simulink model "Collision_two_cars_cs"  (Simulink 8.7)
settings: Solver=ode5  SolverMode=SingleTasking  StartTime=0.0  StopTime=inf  FixedStep=1/20  RelTol=1e-3
model workspace (MAT data in the model file):
  mbox_table.block_array(1).src = 'built-in/Subsystem'
  mbox_table.block_array(1).dest = 'Collision_two_cars_cs/Audi_A8_1'
  mbox_table.block_array(1).mode = 0
  mbox_table.block_array(2).src = 'simulink/Sinks/Out1'
  mbox_table.block_array(2).dest = 'Collision_two_cars_cs/Audi_A8_1/STATE_Audi_A8_1'
  mbox_table.block_array(2).mode = 0
  mbox_table.block_array(3).src = 'PreScanSimulinkLibrary/State'
  mbox_table.block_array(3).dest = 'Collision_two_cars_cs/STATE_Audi_A8_1'
  mbox_table.block_array(3).mode = 0
  mbox_table.block_array(4).src = 'PreScanSimulinkLibrary/Trajectories'
  mbox_table.block_array(4).dest = 'Collision_two_cars_cs/Audi_A8_1/Trajectories'
  mbox_table.block_array(4).mode = 0
  mbox_table.block_array(5).src = 'simulink/Sources/Constant'
  mbox_table.block_array(5).dest = 'Collision_two_cars_cs/Audi_A8_1/Trajectories/Trajectory_1_Offset'
  mbox_table.block_array(5).mode = 0
  mbox_table.block_array(6).src = 'PreScanSimulinkLibrary/Trajectory'
  mbox_table.block_array(6).dest = 'Collision_two_cars_cs/Audi_A8_1/Trajectories/Trajectory_1'
  mbox_table.block_array(6).mode = 0
  mbox_table.block_array(7).src = 'PreScanSimulinkLibrary/Traj2State'
  mbox_table.block_array(7).dest = 'Collision_two_cars_cs/Audi_A8_1/Trajectories/Traj2State1'
  mbox_table.block_array(7).mode = 0
  mbox_table.block_array(8).src = 'simulink/Sinks/Out1'
  mbox_table.block_array(8).dest = 'Collision_two_cars_cs/Audi_A8_1/Trajectories/State'
  mbox_table.block_array(8).mode = 0
  mbox_table.block_array(9).src = 'PreScanSimulinkLibrary/SELF'
  mbox_table.block_array(9).dest = 'Collision_two_cars_cs/SELF_Audi_A8_1'
  mbox_table.block_array(9).mode = 0
  mbox_table.block_array(10).src = 'simulink/Sources/In1'
  mbox_table.block_array(10).dest = 'Collision_two_cars_cs/Audi_A8_1/SELF_Audi_A8_1'
  mbox_table.block_array(10).mode = 0
  mbox_table.block_array(11).src = 'PreScanSimulinkLibrary/DemuxSELF'
  mbox_table.block_array(11).dest = 'Collision_two_cars_cs/Audi_A8_1/SELF_Demux'
  mbox_table.block_array(11).mode = 0
  mbox_table.block_array(12).src = 'built-in/S-Function'
  mbox_table.block_array(12).dest = 'Collision_two_cars_cs/AIR_1'
  mbox_table.block_array(12).mode = 0
  mbox_table.block_array(13).src = 'simulink/Sources/In1'
  mbox_table.block_array(13).dest = 'Collision_two_cars_cs/Audi_A8_1/AIR_1'
  mbox_table.block_array(13).mode = 0
  mbox_table.block_array(14).src = 'PreScanSimulinkLibrary/DemuxAIR'
  mbox_table.block_array(14).dest = 'Collision_two_cars_cs/Audi_A8_1/AIR_1_Demux'
  mbox_table.block_array(14).mode = 0
  mbox_table.block_array(15).src = 'built-in/Subsystem'
  mbox_table.block_array(15).dest = 'Collision_two_cars_cs/BMW_X5_1'
  mbox_table.block_array(15).mode = 0
  mbox_table.block_array(16).src = 'simulink/Sinks/Out1'
  mbox_table.block_array(16).dest = 'Collision_two_cars_cs/BMW_X5_1/STATE_BMW_X5_1'
  mbox_table.block_array(16).mode = 0
  mbox_table.block_array(17).src = 'PreScanSimulinkLibrary/State'
  mbox_table.block_array(17).dest = 'Collision_two_cars_cs/STATE_BMW_X5_1'
  mbox_table.block_array(17).mode = 0
  mbox_table.block_array(18).src = 'PreScanSimulinkLibrary/Trajectories'
  mbox_table.block_array(18).dest = 'Collision_two_cars_cs/BMW_X5_1/Trajectories'
  mbox_table.block_array(18).mode = 0
  mbox_table.block_array(19).src = 'simulink/Sources/Constant'
  mbox_table.block_array(19).dest = 'Collision_two_cars_cs/BMW_X5_1/Trajectories/Trajectory_2_Offset'
  mbox_table.block_array(19).mode = 0
  mbox_table.block_array(20).src = 'PreScanSimulinkLibrary/Trajectory'
  mbox_table.block_array(20).dest = 'Collision_two_cars_cs/BMW_X5_1/Trajectories/Trajectory_2'
  mbox_table.block_array(20).mode = 0
  mbox_table.block_array(21).src = 'PreScanSimulinkLibrary/Traj2State'
  mbox_table.block_array(21).dest = 'Collision_two_cars_cs/BMW_X5_1/Trajectories/Traj2State1'
  mbox_table.block_array(21).mode = 0
  mbox_table.block_array(22).src = 'simulink/Sinks/Out1'
  mbox_table.block_array(22).dest = 'Collision_two_cars_cs/BMW_X5_1/Trajectories/State'
  mbox_table.block_array(22).mode = 0
  mbox_table.block_array(23).src = 'PreScanSimulinkLibrary/SELF'
  mbox_table.block_array(23).dest = 'Collision_two_cars_cs/SELF_BMW_X5_1'
  mbox_table.block_array(23).mode = 0
  mbox_table.block_array(24).src = 'simulink/Sources/In1'
  mbox_table.block_array(24).dest = 'Collision_two_cars_cs/BMW_X5_1/SELF_BMW_X5_1'
  mbox_table.block_array(24).mode = 0
  mbox_table.block_array(25).src = 'PreScanSimulinkLibrary/DemuxSELF'
  mbox_table.block_array(25).dest = 'Collision_two_cars_cs/BMW_X5_1/SELF_Demux'
  mbox_table.block_array(25).mode = 0
  mbox_table.block_array(26).src = 'SimCoreLibrary/SimCoreConfiguration'
  mbox_table.block_array(26).dest = 'Collision_two_cars_cs/SimCoreConfiguration'
  mbox_table.block_array(26).mode = 0
  mbox_table.block_array(27).src = 'SimCoreLibrary/Actuators'
  mbox_table.block_array(27).dest = 'Collision_two_cars_cs/Actuators'
  mbox_table.block_array(27).mode = 0
  mbox_table.block_array(28).src = 'SimCoreLibrary/SetActuators'
  mbox_table.block_array(28).dest = 'Collision_two_cars_cs/SetActuators'
  mbox_table.block_array(28).mode = 0
  mbox_table.block_array(29).src = 'SimCoreLibrary/GetSensors'
  mbox_table.block_array(29).dest = 'Collision_two_cars_cs/GetSensors'
  mbox_table.block_array(29).mode = 0
  mbox_table.block_array(30).src = 'SimCoreLibrary/SimCoreInfo'
  mbox_table.block_array(30).dest = 'Collision_two_cars_cs/SimCoreInfo'
  mbox_table.block_array(30).mode = 0
  mbox_table.block_array(31).src = 'PreScanSimulinkLibrary/Regenerate'
  mbox_table.block_array(31).dest = 'Collision_two_cars_cs/Regenerate'
  mbox_table.block_array(31).mode = 0
  mbox_table.block_array(32).src = 'PreScanSimulinkLibrary/Record for Replay  '
  mbox_table.block_array(32).dest = 'Collision_two_cars_cs/Record for Replay  '
  mbox_table.block_array(32).mode = 0
  mbox_table.block_array(33).src = 'PreScanSimulinkLibrary/Open Useful Blocks'
  mbox_table.block_array(33).dest = 'Collision_two_cars_cs/Open Useful Blocks'
  mbox_table.block_array(33).mode = 0
  mbox_table.block_array(34).src = 'PreScanSimulinkLibrary/PreScan Options   '
  mbox_table.block_array(34).dest = 'Collision_two_cars_cs/PreScan Options   '
  mbox_table.block_array(34).mode = 0
  mbox_table.block_array(35).src = 'built-in/Note'
  mbox_table.block_array(35).dest = 'Collision_two_cars_cs/Version:                  '
  mbox_table.block_array(35).mode = 0
  mbox_table.block_array(36).src = 'built-in/Note'
  mbox_table.block_array(36).dest = 'Collision_two_cars_cs/7.4.0'
  mbox_table.block_array(36).mode = 0
  mbox_table.block_array(37).src = 'built-in/Note'
  mbox_table.block_array(37).dest = 'Collision_two_cars_cs/Author(s):                '
  mbox_table.block_array(37).mode = 0
  mbox_table.block_array(38).src = 'built-in/Note'
  mbox_table.block_array(38).dest = 'Collision_two_cars_cs/Weikas'
  mbox_table.block_array(38).mode = 0
  mbox_table.block_array(39).src = 'built-in/Note'
  mbox_table.block_array(39).dest = 'Collision_two_cars_cs/Descriptive text:      '
  mbox_table.block_array(39).mode = 0
  mbox_table.block_array(40).src = 'built-in/Note'
  mbox_table.block_array(40).dest = 'Collision_two_cars_cs/Collision between two cars'
  mbox_table.block_array(40).mode = 0
  mbox_table.block_array(41).src = 'built-in/Note'
  mbox_table.block_array(41).dest = 'Collision_two_cars_cs/ID
    | 
    | 1
    | 2'
  mbox_table.block_array(41).mode = 0
  mbox_table.block_array(42).src = 'built-in/Note'
  mbox_table.block_array(42).dest = 'Collision_two_cars_cs/OBU-Beacon ID
    | 
    | 
    | '
  mbox_table.block_array(42).mode = 0
  mbox_table.block_array(43).src = 'built-in/Note'
  mbox_table.block_array(43).dest = 'Collision_two_cars_cs/TypeID
    | 
    | 1
    | 1'
  mbox_table.block_array(43).mode = 0
  mbox_table.block_array(44).src = 'built-in/Note'
  mbox_table.block_array(44).dest = 'Collision_two_cars_cs/TypeTag
    | 
    | Car
    | Car'
  mbox_table.block_array(44).mode = 0
  mbox_table.block_array(45).src = 'built-in/Note'
  mbox_table.block_array(45).dest = 'Collision_two_cars_cs/SD
    | 
    | Y
    | Y'
  mbox_table.block_array(45).mode = 0
  mbox_table.block_array(46).src = 'built-in/Note'
  mbox_table.block_array(46).dest = 'Collision_two_cars_cs/CD
    | 
    | N
    | N'
  mbox_table.block_array(46).mode = 0
  mbox_table.block_array(47).src = 'built-in/Note'
  mbox_table.block_array(47).dest = 'Collision_two_cars_cs/Name
    | 
    | Audi_A8_1
    | BMW_X5_1'
  mbox_table.block_array(47).mode = 0
  mbox_table.block_array(48).src = 'built-in/Note'
  mbox_table.block_array(48).dest = 'Collision_two_cars_cs/Num ID       OBU-Beacon ID     Type ID      Type Tag             SD        CD             Name                          '
  mbox_table.block_array(48).mode = 0
  mbox_table.block_array(49).src = 'built-in/Terminator'
  mbox_table.block_array(49).dest = 'Collision_two_cars_cs/BMW_X5_1/Terminator_1'
  mbox_table.block_array(49).mode = 1
  mbox_table.block_array(50).src = 'built-in/Terminator'
  mbox_table.block_array(50).dest = 'Collision_two_cars_cs/BMW_X5_1/Terminator_2'
  mbox_table.block_array(50).mode = 1
  mbox_table.block_array(51).src = 'built-in/Terminator'
  mbox_table.block_array(51).dest = 'Collision_two_cars_cs/BMW_X5_1/Terminator_3'
  mbox_table.block_array(51).mode = 1
  mbox_table.block_array(52).src = 'built-in/Terminator'
  mbox_table.block_array(52).dest = 'Collision_two_cars_cs/BMW_X5_1/Terminator_4'
  mbox_table.block_array(52).mode = 1
  mbox_table.block_array(53).src = 'built-in/Terminator'
  mbox_table.block_array(53).dest = 'Collision_two_cars_cs/BMW_X5_1/Terminator_5'
  mbox_table.block_array(53).mode = 1
  mbox_table.block_array(54).src = 'built-in/Terminator'
  mbox_table.block_array(54).dest = 'Collision_two_cars_cs/BMW_X5_1/Terminator_6'
  mbox_table.block_array(54).mode = 1
  mbox_table.block_array(55).src = 'built-in/Terminator'
  mbox_table.block_array(55).dest = 'Collision_two_cars_cs/BMW_X5_1/Terminator_7'
  mbox_table.block_array(55).mode = 1
  mbox_table.block_array(56).src = 'built-in/Terminator'
  mbox_table.block_array(56).dest = 'Collision_two_cars_cs/BMW_X5_1/Terminator_8'
  mbox_table.block_array(56).mode = 1
  mbox_table.block_array(57).src = 'built-in/Terminator'
  mbox_table.block_array(57).dest = 'Collision_two_cars_cs/BMW_X5_1/Terminator_9'
  mbox_table.block_array(57).mode = 1
  mbox_table.block_array(58).src = 'built-in/Terminator'
  mbox_table.block_array(58).dest = 'Collision_two_cars_cs/BMW_X5_1/Terminator_10'
  mbox_table.block_array(58).mode = 1
  mbox_table.block_array(59).src = 'built-in/Terminator'
  mbox_table.block_array(59).dest = 'Collision_two_cars_cs/BMW_X5_1/Terminator_11'
  mbox_table.block_array(59).mode = 1
  mbox_table.block_array(60).src = 'built-in/Terminator'
  mbox_table.block_array(60).dest = 'Collision_two_cars_cs/BMW_X5_1/Terminator_12'
  mbox_table.block_array(60).mode = 1
  mbox_table.block_index : java.util.Hashtable (value not decoded)
  mbox_table.line_array(1).sys = 'Collision_two_cars_cs'
  mbox_table.line_array(1).line_id = 'L1'
  mbox_table.line_array(1).iport = 'STATE_Audi_A8_1/1'
  mbox_table.line_array(1).oport = 'Audi_A8_1/1'
  mbox_table.line_array(1).mode = 0
  mbox_table.line_array(2).sys = 'Collision_two_cars_cs/Audi_A8_1/Trajectories'
  mbox_table.line_array(2).line_id = 'L2'
  mbox_table.line_array(2).iport = 'Traj2State1/1'
  mbox_table.line_array(2).oport = 'Trajectory_1/1'
  mbox_table.line_array(2).mode = 0
  mbox_table.line_array(3).sys = 'Collision_two_cars_cs/Audi_A8_1/Trajectories'
  mbox_table.line_array(3).line_id = 'L3'
  mbox_table.line_array(3).iport = 'Traj2State1/2'
  mbox_table.line_array(3).oport = 'Trajectory_1_Offset/1'
  mbox_table.line_array(3).mode = 0
  mbox_table.line_array(4).sys = 'Collision_two_cars_cs/Audi_A8_1/Trajectories'
  mbox_table.line_array(4).line_id = 'L4'
  mbox_table.line_array(4).iport = 'State/1'
  mbox_table.line_array(4).oport = 'Traj2State1/1'
  mbox_table.line_array(4).mode = 0
  mbox_table.line_array(5).sys = 'Collision_two_cars_cs'
  mbox_table.line_array(5).line_id = 'L5'
  mbox_table.line_array(5).iport = 'Audi_A8_1/1'
  mbox_table.line_array(5).oport = 'SELF_Audi_A8_1/1'
  mbox_table.line_array(5).mode = 0
  mbox_table.line_array(6).sys = 'Collision_two_cars_cs/Audi_A8_1'
  mbox_table.line_array(6).line_id = 'L6'
  mbox_table.line_array(6).iport = 'SELF_Demux/1'
  mbox_table.line_array(6).oport = 'SELF_Audi_A8_1/1'
  mbox_table.line_array(6).mode = 0
  mbox_table.line_array(7).sys = 'Collision_two_cars_cs/Audi_A8_1'
  mbox_table.line_array(7).line_id = 'L7'
  mbox_table.line_array(7).iport = 'AIR_1_Demux/1'
  mbox_table.line_array(7).oport = 'AIR_1/1'
  mbox_table.line_array(7).mode = 0
  mbox_table.line_array(8).sys = 'Collision_two_cars_cs'
  mbox_table.line_array(8).line_id = 'L8'
  mbox_table.line_array(8).iport = 'Audi_A8_1/2'
  mbox_table.line_array(8).oport = 'AIR_1/1'
  mbox_table.line_array(8).mode = 0
  mbox_table.line_array(9).sys = 'Collision_two_cars_cs/Audi_A8_1'
  mbox_table.line_array(9).line_id = 'L9'
  mbox_table.line_array(9).iport = 'STATE_Audi_A8_1/1'
  mbox_table.line_array(9).oport = 'Trajectories/1'
  mbox_table.line_array(9).mode = 0
  mbox_table.line_array(10).sys = 'Collision_two_cars_cs'
  mbox_table.line_array(10).line_id = 'L10'
  mbox_table.line_array(10).iport = 'STATE_BMW_X5_1/1'
  mbox_table.line_array(10).oport = 'BMW_X5_1/1'
  mbox_table.line_array(10).mode = 0
  mbox_table.line_array(11).sys = 'Collision_two_cars_cs/BMW_X5_1/Trajectories'
  mbox_table.line_array(11).line_id = 'L11'
  mbox_table.line_array(11).iport = 'Traj2State1/1'
  mbox_table.line_array(11).oport = 'Trajectory_2/1'
  mbox_table.line_array(11).mode = 0
  mbox_table.line_array(12).sys = 'Collision_two_cars_cs/BMW_X5_1/Trajectories'
  mbox_table.line_array(12).line_id = 'L12'
  mbox_table.line_array(12).iport = 'Traj2State1/2'
  mbox_table.line_array(12).oport = 'Trajectory_2_Offset/1'
  mbox_table.line_array(12).mode = 0
  mbox_table.line_array(13).sys = 'Collision_two_cars_cs/BMW_X5_1/Trajectories'
  mbox_table.line_array(13).line_id = 'L13'
  mbox_table.line_array(13).iport = 'State/1'
  mbox_table.line_array(13).oport = 'Traj2State1/1'
  mbox_table.line_array(13).mode = 0
  mbox_table.line_array(14).sys = 'Collision_two_cars_cs'
  mbox_table.line_array(14).line_id = 'L14'
  mbox_table.line_array(14).iport = 'BMW_X5_1/1'
  mbox_table.line_array(14).oport = 'SELF_BMW_X5_1/1'
  mbox_table.line_array(14).mode = 0
  mbox_table.line_array(15).sys = 'Collision_two_cars_cs/BMW_X5_1'
  mbox_table.line_array(15).line_id = 'L15'
  mbox_table.line_array(15).iport = 'SELF_Demux/1'
  mbox_table.line_array(15).oport = 'SELF_BMW_X5_1/1'
  mbox_table.line_array(15).mode = 0
  mbox_table.line_array(16).sys = 'Collision_two_cars_cs/BMW_X5_1'
  mbox_table.line_array(16).line_id = 'L16'
  mbox_table.line_array(16).iport = 'STATE_BMW_X5_1/1'
  mbox_table.line_array(16).oport = 'Trajectories/1'
  mbox_table.line_array(16).mode = 0
  mbox_table.line_array(17).sys = 'Collision_two_cars_cs/BMW_X5_1'
  mbox_table.line_array(17).line_id = 'l1'
  mbox_table.line_array(17).iport = 'Terminator_1/1'
  mbox_table.line_array(17).oport = 'SELF_Demux/1'
  mbox_table.line_array(17).mode = 1
  mbox_table.line_array(18).sys = 'Collision_two_cars_cs/BMW_X5_1'
  mbox_table.line_array(18).line_id = 'l2'
  mbox_table.line_array(18).iport = 'Terminator_2/1'
  mbox_table.line_array(18).oport = 'SELF_Demux/2'
  mbox_table.line_array(18).mode = 1
  mbox_table.line_array(19).sys = 'Collision_two_cars_cs/BMW_X5_1'
  mbox_table.line_array(19).line_id = 'l3'
  mbox_table.line_array(19).iport = 'Terminator_3/1'
  mbox_table.line_array(19).oport = 'SELF_Demux/3'
  mbox_table.line_array(19).mode = 1
  mbox_table.line_array(20).sys = 'Collision_two_cars_cs/BMW_X5_1'
  mbox_table.line_array(20).line_id = 'l4'
  mbox_table.line_array(20).iport = 'Terminator_4/1'
  mbox_table.line_array(20).oport = 'SELF_Demux/4'
  mbox_table.line_array(20).mode = 1
  mbox_table.line_array(21).sys = 'Collision_two_cars_cs/BMW_X5_1'
  mbox_table.line_array(21).line_id = 'l5'
  mbox_table.line_array(21).iport = 'Terminator_5/1'
  mbox_table.line_array(21).oport = 'SELF_Demux/5'
  mbox_table.line_array(21).mode = 1
  mbox_table.line_array(22).sys = 'Collision_two_cars_cs/BMW_X5_1'
  mbox_table.line_array(22).line_id = 'l6'
  mbox_table.line_array(22).iport = 'Terminator_6/1'
  mbox_table.line_array(22).oport = 'SELF_Demux/6'
  mbox_table.line_array(22).mode = 1
  mbox_table.line_array(23).sys = 'Collision_two_cars_cs/BMW_X5_1'
  mbox_table.line_array(23).line_id = 'l7'
  mbox_table.line_array(23).iport = 'Terminator_7/1'
  mbox_table.line_array(23).oport = 'SELF_Demux/7'
  mbox_table.line_array(23).mode = 1
  mbox_table.line_array(24).sys = 'Collision_two_cars_cs/BMW_X5_1'
  mbox_table.line_array(24).line_id = 'l8'
  mbox_table.line_array(24).iport = 'Terminator_8/1'
  mbox_table.line_array(24).oport = 'SELF_Demux/8'
  mbox_table.line_array(24).mode = 1
  mbox_table.line_array(25).sys = 'Collision_two_cars_cs/BMW_X5_1'
  mbox_table.line_array(25).line_id = 'l9'
  mbox_table.line_array(25).iport = 'Terminator_9/1'
  mbox_table.line_array(25).oport = 'SELF_Demux/9'
  mbox_table.line_array(25).mode = 1
  mbox_table.line_array(26).sys = 'Collision_two_cars_cs/BMW_X5_1'
  mbox_table.line_array(26).line_id = 'l10'
  mbox_table.line_array(26).iport = 'Terminator_10/1'
  mbox_table.line_array(26).oport = 'SELF_Demux/10'
  mbox_table.line_array(26).mode = 1
  mbox_table.line_array(27).sys = 'Collision_two_cars_cs/BMW_X5_1'
  mbox_table.line_array(27).line_id = 'l11'
  mbox_table.line_array(27).iport = 'Terminator_11/1'
  mbox_table.line_array(27).oport = 'SELF_Demux/11'
  mbox_table.line_array(27).mode = 1
  mbox_table.line_array(28).sys = 'Collision_two_cars_cs/BMW_X5_1'
  mbox_table.line_array(28).line_id = 'l12'
  mbox_table.line_array(28).iport = 'Terminator_12/1'
  mbox_table.line_array(28).oport = 'SELF_Demux/12'
  mbox_table.line_array(28).mode = 1
  mbox_table.line_index : java.util.Hashtable (value not decoded)
  mbox_table.next_linenr = 17
  mbox_table.next_termlinenr = 13
  model_closed = 0
  sim_status = 0
PreLoadFcn:
  | check_NUTS_defined;
  | 
  | assignin('base',['model_closed_' bdroot],false);
InitFcn:
  | PreScanExperimentInitFcn(bdroot)
StopFcn:
  | PreScanExperimentStopFcn(bdroot)
libraries: PreScanSimulinkLibrary x8, PreScanUsefulBlocks x2
(part 1 of 2)
CloseFcn:
  | evalin('base',['clear model_closed_' bdroot]);
settings Model: Creator=PRESCAN  LastModifiedBy=agrawal  SnapshotBufferSize=1000
settings DataIOCC: SignalLoggingSaveFormat=ModelDataLogs
settings OptimizationCC: ExpressionDepthLimit=2147483647  InitFltsAndDblsToZero=on
settings DebuggingCC: SaveWithParameterizedLinksMsg=none  SignalResolutionControl=TryResolveAllWithWarning  MultiTaskDSMMsg=warning  MultiTaskCondExecSysMsg=none  FcnCallInpInsideContextMsg=UseLocalSettings  StateNameClashWarn=warning
settings GRTTargetCC: TargetFcnLib=ansi_tfl_tmw.mat  CombineOutputUpdateFcns=off  GRTInterface=on

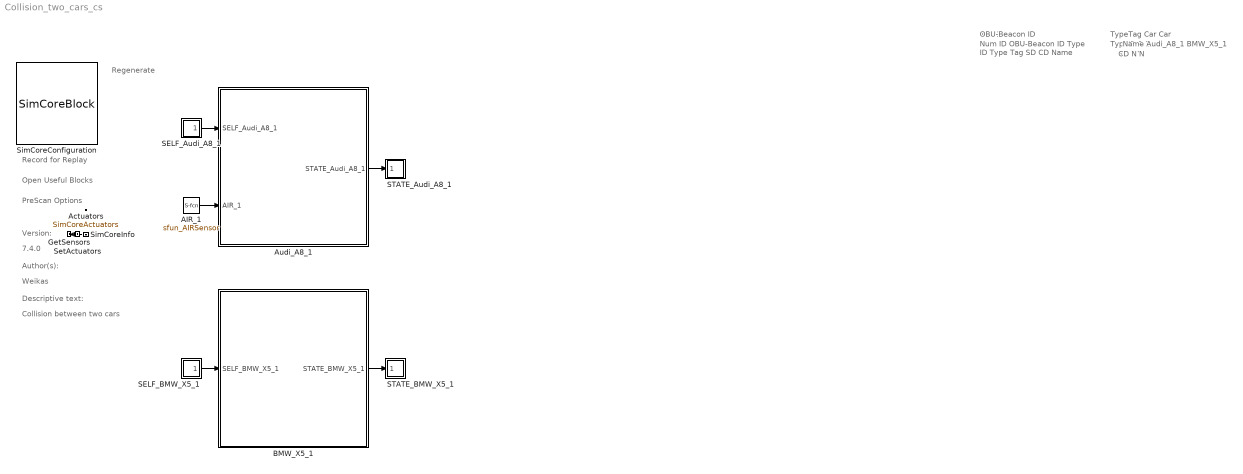
== system Collision_two_cars_cs ==
  note: Regenerate
  note: Record for Replay
  note: Open Useful Blocks
  note: PreScan Options
  note: Version:
  note: 7.4.0
  note: Author(s):
  note: Weikas
  note: Descriptive text:
  note: Collision between two cars
  note: Num ID OBU-Beacon ID Type ID Type Tag SD CD Name
  note: ID
      |
      | 1
      | 2
  note: OBU-Beacon ID
  note: TypeID
      |
      | 1
      | 1
  note: TypeTag
      |
      | Car
      | Car
  note: SD
      |
      | Y
      | Y
  note: CD
      |
      | N
      | N
  note: Name
      |
      | Audi_A8_1
      | BMW_X5_1
  AIR_1 : S-Function  Priority=3  LoadFcn=load('PrescanAIRSensorData.mat');load('PrescanAIRSensorMessage.mat')  FunctionName=sfun_AIRSensor  Parameters=timestepMask maxInputMessages maxOutputMessages sensorID detectableObjects  SFunctionDeploymentMode=off  EnableBusSupport=off  mask{timestepMask=1/20, maxInputMessages=0, maxOutputMessages=1, sensorID=161, detectableObjects=1}
      mask prompts: timestepMask "MATLAB timestep:"; maxInputMessages "Max input messages:"; maxOutputMessages "Max output messages:"; sensorID "Sensor ID:"; detectableObjects "Max detectable objects:"
      mask help: AIR sensor I/O
      mask Display: image(imread('AIR.png'))
  Actuators : DataStoreMemory  DataStoreName=SimCoreActuators  InitialValue=zeros(30,1)  ShowAdditionalParam=off
  Audi_A8_1 : Subsystem  Tag=WorldObjectSubSystem  InitFcn=UniqueId = '152';
      mask Display: image(imread('Audi_A8.jpg'));color('white');text(0,0,' ID=1\n')
  BMW_X5_1 : Subsystem  Tag=WorldObjectSubSystem  InitFcn=UniqueId = '158';
      mask Display: image(imread('BMW_X5.jpg'));color('white');text(0,0,' ID=2\n')
  GetSensors : Subsystem  Tag=GetSensors  Priority=2  mask(PreScan Simulation Core Block){NrOfSensors=22, TimeStep=1/20}
      mask prompts: NrOfSensors "Number of sensor values"; TimeStep "Timestep [s]"
      mask help:
      | Please do not remove this block from the PreScan compilation sheet,
      | as it contains essential configuration parameters for a PreScan simulation.
      settings: DeleteFcn=PreScanBlockDeleteFcn;
  SELF_Audi_A8_1 : Subsystem  Tag=SELF  Priority=3  mask(PreScan Source Block: SELF){PortName=SELF_Audi_A8_1, PortIndex=0, PortWidth=8, TimeStep=1/20}
      mask prompts: PortName "Auto-Assigned: Port Name [-]"; PortIndex "Auto-Assigned: Port Index [-]"; PortWidth "Auto-Assigned: Port Dimensions"; TimeStep "Auto-Assigned: Upload Period [s]"
      mask help:
      | The SELF port shows (state) information of the actor itself. The outputs are position in the experiment's axis system and the GPS coordinates, and the object's absolute velocity and compass heading.
      |
      | For more information, please click Help.
      settings: DeleteFcn=PreScanBlockDeleteFcn;
      mask Help: eval('openHelp(462)')
      mask Display: image(imread('GPS.png'))
  SELF_BMW_X5_1 : Subsystem  Tag=SELF  Priority=3  mask(PreScan Source Block: SELF){PortName=SELF_BMW_X5_1, PortIndex=14, PortWidth=8, TimeStep=1/20}
      mask prompts: PortName "Auto-Assigned: Port Name [-]"; PortIndex "Auto-Assigned: Port Index [-]"; PortWidth "Auto-Assigned: Port Dimensions"; TimeStep "Auto-Assigned: Upload Period [s]"
      mask help:
      | The SELF port shows (state) information of the actor itself. The outputs are position in the experiment's axis system and the GPS coordinates, and the object's absolute velocity and compass heading.
      |
      | For more information, please click Help.
      settings: DeleteFcn=PreScanBlockDeleteFcn;
      mask Help: eval('openHelp(462)')
      mask Display: image(imread('GPS.png'))
  STATE_Audi_A8_1 : Subsystem  Tag=State  Priority=0  mask(PreScan Sink Block: State){x0=377.900390625, y0=-8.5285453796386719, z0=0.55, Roll0=0, Pitch0=0, Yaw0=0, TimeStep=1/20}
      mask prompts: x0 "Ini x-position VEHICLE wrt GLOBAL axis system [m]"; y0 "Ini y-position VEHICLE wrt GLOBAL axis system [m]"; z0 "Ini z-position VEHICLE wrt GLOBAL axis system [m]"; Roll0 "Ini roll-angle BODY wrt VEHICLE axis system [deg]"; Pitch0 "Ini pitch-angle BODY wrt VEHICLE axis system [deg]"; Yaw0 "Ini yaw-angle VEHICLE wrt GLOBAL axis system [deg]"; TimeStep "Time Step [s]"
      mask help:
      | The Actor State contains a vector signal of size (9x1), containing the following signals:
      |
      | -  Position                  (x,y,z)                                     [m]
      | -  Velocity                  (vx,vy,vz)                               [m/s]
      | -  Angles                    (Roll, Pitch, Yaw)                   [rad]
      |
      | The Actor state is defined in the global axis system.
      | The state is superponed on the Initial position defined in the GUI.
      |
      | For more information, please click Help.
      settings: DeleteFcn=PreScanBlockDeleteFcn;
      mask Help: eval('openHelp(222)')
      mask Display: image(imread('State.png'))
  STATE_BMW_X5_1 : Subsystem  Tag=State  Priority=0  mask(PreScan Sink Block: State){x0=479.06998617115, y0=3.3927311126021005, z0=0.69, Roll0=0, Pitch0=0, Yaw0=131.5594047339099, TimeStep=1/20}
      mask prompts: x0 "Ini x-position VEHICLE wrt GLOBAL axis system [m]"; y0 "Ini y-position VEHICLE wrt GLOBAL axis system [m]"; z0 "Ini z-position VEHICLE wrt GLOBAL axis system [m]"; Roll0 "Ini roll-angle BODY wrt VEHICLE axis system [deg]"; Pitch0 "Ini pitch-angle BODY wrt VEHICLE axis system [deg]"; Yaw0 "Ini yaw-angle VEHICLE wrt GLOBAL axis system [deg]"; TimeStep "Time Step [s]"
      mask help:
      | The Actor State contains a vector signal of size (9x1), containing the following signals:
      |
      | -  Position                  (x,y,z)                                     [m]
      | -  Velocity                  (vx,vy,vz)                               [m/s]
      | -  Angles                    (Roll, Pitch, Yaw)                   [rad]
      |
      | The Actor state is defined in the global axis system.
      | The state is superponed on the Initial position defined in the GUI.
      |
      | For more information, please click Help.
      settings: DeleteFcn=PreScanBlockDeleteFcn;
      mask Help: eval('openHelp(222)')
      mask Display: image(imread('State.png'))
  SetActuators : Subsystem  Tag=SetActuators  Priority=1  mask(PreScan Simulation Core Block){TimeStep=1/20, NrOfActuators=30}
      mask prompts: TimeStep "Timestep [s]"; NrOfActuators "Number of actuator values"
      mask help:
      | Please do not remove this block from the PreScan compilation sheet,
      | as it contains essential configuration parameters for a PreScan simulation.
      settings: DeleteFcn=PreScanBlockDeleteFcn;
  SimCoreConfiguration : M-S-Function  Tag=SimCoreConfiguration  Description=123BB2F9386A806AF0CDF74150241FF776EE166490DEEAC00F97687BB92383BD  FunctionName=SimCoreBlock  Parameters=ExperimentXML PortsXML SimulationCore HostName CheckStart EnableLog RfR EnableGPUAccel ShowComputationTime  mask(PreScan Simulation Core Configurator){SimulationCore=NUTS, HostName=0, CheckStart=0, prescanversion='7.4.0', EnableLog=off, RfR=0, EnableGPUAccel=off, ShowComputationTime=off}
      mask prompts: SimulationCore "Simulation Core"; HostName "Simulation Host"; CheckStart "Show START Dialog"; prescanversion "PreScan Version"; EnableLog "Create TA Log"; RfR "Record for Replay"; EnableGPUAccel "Enable GPU Acceleration"; ShowComputationTime "Show ComputationTime Scope"
      mask help:
      | Please do not remove this block from the PreScan compilation sheet,
      | as it contains essential configuration parameter for a PreScan simulation.
      mask init:
      | model = bdroot;
      | ExperimentXML = [model(1:end-3) '.pex'];
      | PortsXML = [model '_ports.pcd'];
      settings: DeleteFcn=PreScanBlockDeleteFcn;  ModelCloseFcn=assignin('base',['model_closed_' bdroot],true);
      mask Help: eval('openHelp(812)')
      mask Display: image(imread('prescanlogo.ico'))
  SimCoreInfo : Subsystem  Tag=SimCoreInfo
  wires:
  SetActuators/1(dummy) -> GetSensors/1(dummy)
  Audi_A8_1/1(STATE_Audi_A8_1) -> STATE_Audi_A8_1/1(State)
  SELF_Audi_A8_1/1(U) -> Audi_A8_1/1(SELF_Audi_A8_1)
  AIR_1/1 -> Audi_A8_1/2(AIR_1)
  BMW_X5_1/1(STATE_BMW_X5_1) -> STATE_BMW_X5_1/1(State)
  SELF_BMW_X5_1/1(U) -> BMW_X5_1/1(SELF_BMW_X5_1)

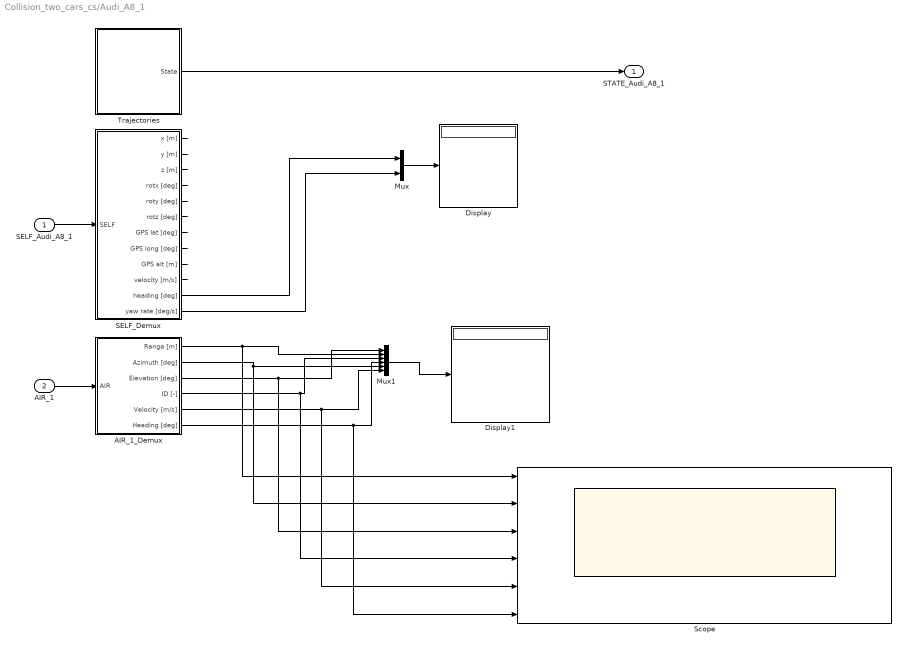
== system Collision_two_cars_cs/Audi_A8_1 ==
  SELF_Audi_A8_1 : Inport  Tag=SELFInport
  AIR_1 : Inport  Tag=AIRInport  Port=2  OutDataTypeStr=Bus: PRESCAN_AIRSENSORMESSAGE
  AIR_1_Demux : Subsystem  Tag=DemuxAIR  mask(PreScan Demux Block: AIR){DetectionType=BBox, detectableObjects=1}
      mask prompts: DetectionType "Detection Type"; detectableObjects "Max. detectable objects"
      mask help:
      | The Actor Information Receiver sensor provides a fast, simple and generic detection solution which is not tied up to a specific technology and can be used for scenarios in which a simple sensor is needed.
      |
      | For more information, please click Help.
      mask init:
      | switch DetectionType
      |     case 1
      |         DetectionTypeStr = 'Center';
      |     case 2
      |         DetectionTypeStr = 'BBox';
      |     case 3
      |         DetectionTypeStr = 'CoG';
      |     otherwise
      |         DetectionTypeStr = 'Unknown';
      | end
      settings: DeleteFcn=PreScanBlockDeleteFcn;
      mask Help: eval('openHelp(411)')
      mask TypeOptions DetectionType: Center | BBox | CoG
      mask Display:
      | disp(char('Det. type:         ',['{\it',DetectionTypeStr,'}']),'texmode','on')
      | port_label('output',1,'Range [m]')
      | port_label('output',2,'{\theta} [deg]','texmode','on')
      | port_label('output',3,'{\phi} [deg]','texmode','on')
      | port_label('output',4,'ID [-]','texmode','on')
      | port_label('output',5,'Velocity [m/s]','texmode','on')
      | port_label('output',6,'Heading [deg]','texmode','on')
  Display : Display
  Display1 : Display
  Mux : Mux  Inputs=2
      settings: DisplayOption=signals
  Mux1 : Mux  Inputs=6
      settings: DisplayOption=signals
  SELF_Demux : Subsystem  Tag=DemuxSELF  mask(PreScan Demux Block:){}
      settings: DeleteFcn=PreScanBlockDeleteFcn;
      mask Display:
      | port_label('output',1,'x [m]')
      | port_label('output',2,'y [m]')
      | port_label('output',3,'z [m]','texmode','on')
      | port_label('output',4,'Rotx [deg]','texmode','on')
      | port_label('output',5,'Roty [deg]','texmode','on')
      | port_label('output',6,'Rotz [deg]','texmode','on')
      | port_label('output',7,'GPS lat [deg]','texmode','on')
      | port_label('output',8,'GPS long [deg]','texmode','on')
      | port_label('output',9,'GPS alt [m]','texmode','on')
      | port_label('output',10,'Velocity [m/s]')
      | port_label('output',11,'Heading [deg]')
      | port_label('output',12,'Yaw rate [deg/s]')
  Scope : Scope  NumInputPorts=6
  Trajectories : Subsystem  Tag=Trajectories  mask(PreScan Source Block: Trajectories){}
      mask help:
      | The Trajectory block contains the trajectories defined in the PreScan Experiment Editor. The output of the trajectory block is the (vehicle) State.
      |
      | For more information, please click Help.
      settings: DeleteFcn=PreScanBlockDeleteFcn;
      mask Help: eval('openHelp(312)')
      mask Display: image(imread('Trajectory.png'));
  STATE_Audi_A8_1 : Outport  Tag=StateOutport
  wires:
  SELF_Demux/1(x [m]) -> ?
  SELF_Demux/2(y [m]) -> ?
  SELF_Demux/3(z [m]) -> ?
  SELF_Demux/4(rotx [deg]) -> ?
  SELF_Demux/5(roty [deg]) -> ?
  SELF_Demux/6(rotz [deg]) -> ?
  SELF_Demux/7(GPS lat [deg]) -> ?
  SELF_Demux/8(GPS long [deg]) -> ?
  SELF_Demux/9(GPS alt [m]) -> ?
  SELF_Demux/10(velocity [m/s]) -> ?
  SELF_Demux/11(heading [deg]) -> Mux/1
  SELF_Demux/12(yaw rate [deg/s]) -> Mux/2
  Mux/1 -> Display/1
  Mux1/1 -> Display1/1
  AIR_1_Demux/1(Range [m]) -> Scope/1, Mux1/2
  AIR_1_Demux/2(Azimuth [deg]) -> Scope/2, Mux1/5
  AIR_1_Demux/3(Elevation [deg]) -> Scope/3, Mux1/1
  AIR_1_Demux/4(ID [-]) -> Scope/4, Mux1/3
  AIR_1_Demux/5(Velocity [m/s]) -> Scope/5, Mux1/6
  AIR_1_Demux/6(Heading [deg]) -> Scope/6, Mux1/4
  SELF_Audi_A8_1/1 -> SELF_Demux/1(SELF)
  AIR_1/1 -> AIR_1_Demux/1(AIR)
  Trajectories/1(State) -> STATE_Audi_A8_1/1

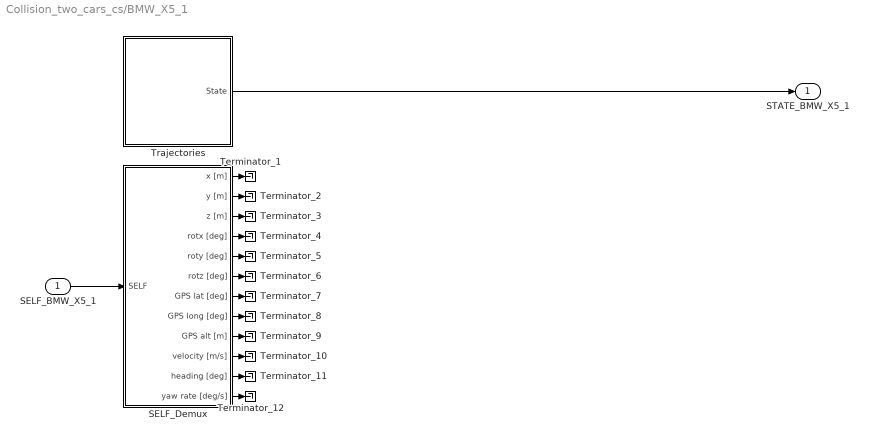
== system Collision_two_cars_cs/BMW_X5_1 ==
  SELF_BMW_X5_1 : Inport  Tag=SELFInport
  SELF_Demux : Subsystem  Tag=DemuxSELF  mask(PreScan Demux Block:){}
      settings: DeleteFcn=PreScanBlockDeleteFcn;
      mask Display:
      | port_label('output',1,'x [m]')
      | port_label('output',2,'y [m]')
      | port_label('output',3,'z [m]','texmode','on')
      | port_label('output',4,'Rotx [deg]','texmode','on')
      | port_label('output',5,'Roty [deg]','texmode','on')
      | port_label('output',6,'Rotz [deg]','texmode','on')
      | port_label('output',7,'GPS lat [deg]','texmode','on')
      | port_label('output',8,'GPS long [deg]','texmode','on')
      | port_label('output',9,'GPS alt [m]','texmode','on')
      | port_label('output',10,'Velocity [m/s]')
      | port_label('output',11,'Heading [deg]')
      | port_label('output',12,'Yaw rate [deg/s]')
  Terminator_{1..12} (12 alike) : Terminator
  Trajectories : Subsystem  Tag=Trajectories  mask(PreScan Source Block: Trajectories){}
      mask help:
      | The Trajectory block contains the trajectories defined in the PreScan Experiment Editor. The output of the trajectory block is the (vehicle) State.
      |
      | For more information, please click Help.
      settings: DeleteFcn=PreScanBlockDeleteFcn;
      mask Help: eval('openHelp(312)')
      mask Display: image(imread('Trajectory.png'));
  STATE_BMW_X5_1 : Outport  Tag=StateOutport
  wires:
  SELF_BMW_X5_1/1 -> SELF_Demux/1(SELF)
  Trajectories/1(State) -> STATE_BMW_X5_1/1
  SELF_Demux/1(x [m]) -> Terminator_1/1
  SELF_Demux/2(y [m]) -> Terminator_2/1
  SELF_Demux/3(z [m]) -> Terminator_3/1
  SELF_Demux/4(rotx [deg]) -> Terminator_4/1
  SELF_Demux/5(roty [deg]) -> Terminator_5/1
  SELF_Demux/6(rotz [deg]) -> Terminator_6/1
  SELF_Demux/7(GPS lat [deg]) -> Terminator_7/1
  SELF_Demux/8(GPS long [deg]) -> Terminator_8/1
  SELF_Demux/9(GPS alt [m]) -> Terminator_9/1
  SELF_Demux/10(velocity [m/s]) -> Terminator_10/1
  SELF_Demux/11(heading [deg]) -> Terminator_11/1
  SELF_Demux/12(yaw rate [deg/s]) -> Terminator_12/1

== system Collision_two_cars_cs/GetSensors ==
  dummy : Inport
  GetSensors : M-S-Function  FunctionName=GetSensorsBlock  Parameters=TimeStep NrOfSensors
  tag scope: SimCoreSensors=global
  wires:
  GetSensors/1 -> [SimCoreSensors]
  dummy/1 -> GetSensors/1

== system Collision_two_cars_cs/SELF_Audi_A8_1 ==
  Selector : Selector  IndexMode=Zero-based  IndexOptions=Starting index (dialog)  Indices=PortIndex  OutputSizes=PortWidth(1)
  U : Outport
  wires:
  Selector/1 -> U/1
  [SimCoreSensors] -> Selector/1

== system Collision_two_cars_cs/SELF_BMW_X5_1 ==
  Selector : Selector  IndexMode=Zero-based  IndexOptions=Starting index (dialog)  Indices=PortIndex  OutputSizes=PortWidth(1)
  U : Outport
  wires:
  Selector/1 -> U/1
  [SimCoreSensors] -> Selector/1

== system Collision_two_cars_cs/STATE_Audi_A8_1 ==
  State : Inport  SampleTime=TimeStep
  Acceleration : Subsystem  mask(ToSensorWorld){PortName=Acceleration_Audi_A8_1, PortIndex=6, PortWidth=3, TimeStep=1/20}
      mask prompts: PortName "Port Name [-]"; PortIndex "Index [-]"; PortWidth "Port Dimensions [-]"; TimeStep "Upload Period [s]"
      mask help: Sends signal(s) from Simulink to the Sensor World
      mask Help:
      | Sends signal(s) from Simulink to the Sensor World.
      | 
      | - Port Name [-]: specifies the name of the output terminal of the Simulink block.
      | - Index [-]: specifies the start position in the output vector sent to the Sensor World
      | - Port dimensions [-]: specifies the width (number of scalars) of the output port
      | - Upload period [s]: specifies the upload period (in seconds) of the port.
      mask Display: port_label('input', 1, PortName)
  Demux : Demux  Outputs=5
  Position : Subsystem  mask(ToSensorWorld){PortName=Position_Audi_A8_1, PortIndex=0, PortWidth=3, TimeStep=1/20}
      mask prompts: PortName "Port Name [-]"; PortIndex "Index [-]"; PortWidth "Port Dimensions [-]"; TimeStep "Upload Period [s]"
      mask help: Sends signal(s) from Simulink to the Sensor World
      mask Help:
      | Sends signal(s) from Simulink to the Sensor World.
      | 
      | - Port Name [-]: specifies the name of the output terminal of the Simulink block.
      | - Index [-]: specifies the start position in the output vector sent to the Sensor World
      | - Port dimensions [-]: specifies the width (number of scalars) of the output port
      | - Upload period [s]: specifies the upload period (in seconds) of the port.
      mask Display: port_label('input', 1, PortName)
  RPY : Subsystem  mask(ToSensorWorld){PortName=RPY_Audi_A8_1, PortIndex=9, PortWidth=3, TimeStep=1/20}
      mask prompts: PortName "Port Name [-]"; PortIndex "Index [-]"; PortWidth "Port Dimensions [-]"; TimeStep "Upload Period [s]"
      mask help: Sends signal(s) from Simulink to the Sensor World
      mask Help:
      | Sends signal(s) from Simulink to the Sensor World.
      | 
      | - Port Name [-]: specifies the name of the output terminal of the Simulink block.
      | - Index [-]: specifies the start position in the output vector sent to the Sensor World
      | - Port dimensions [-]: specifies the width (number of scalars) of the output port
      | - Upload period [s]: specifies the upload period (in seconds) of the port.
      mask Display: port_label('input', 1, PortName)
  Velocity : Subsystem  mask(ToSensorWorld){PortName=Velocity_Audi_A8_1, PortIndex=3, PortWidth=3, TimeStep=1/20}
      mask prompts: PortName "Port Name [-]"; PortIndex "Index [-]"; PortWidth "Port Dimensions [-]"; TimeStep "Upload Period [s]"
      mask help: Sends signal(s) from Simulink to the Sensor World
      mask Help:
      | Sends signal(s) from Simulink to the Sensor World.
      | 
      | - Port Name [-]: specifies the name of the output terminal of the Simulink block.
      | - Index [-]: specifies the start position in the output vector sent to the Sensor World
      | - Port dimensions [-]: specifies the width (number of scalars) of the output port
      | - Upload period [s]: specifies the upload period (in seconds) of the port.
      mask Display: port_label('input', 1, PortName)
  iniBODYAngles wrtVEH [rad] : Constant  Value=[Roll0 Pitch0 0]  SampleTime=TimeStep
  iniVEHAngles wrtGLOB [rad] : Constant  Value=[0 0 Yaw0]  SampleTime=TimeStep
  iniVEHposition wrtGLOB [m] : Constant  Value=[x0 y0 z0]  SampleTime=TimeStep
  state2FullState : PreScanSimulinkLibrary/state2FullState  SystemSampleTime=-1
  velRPY : Subsystem  mask(ToSensorWorld){PortName=velRPY_Audi_A8_1, PortIndex=12, PortWidth=3, TimeStep=1/20}
      mask prompts: PortName "Port Name [-]"; PortIndex "Index [-]"; PortWidth "Port Dimensions [-]"; TimeStep "Upload Period [s]"
      mask help: Sends signal(s) from Simulink to the Sensor World
      mask Help:
      | Sends signal(s) from Simulink to the Sensor World.
      | 
      | - Port Name [-]: specifies the name of the output terminal of the Simulink block.
      | - Index [-]: specifies the start position in the output vector sent to the Sensor World
      | - Port dimensions [-]: specifies the width (number of scalars) of the output port
      | - Upload period [s]: specifies the upload period (in seconds) of the port.
      mask Display: port_label('input', 1, PortName)
  wires:
  Demux/5 -> velRPY/1(Y)
  Demux/4 -> RPY/1(Y)
  Demux/3 -> Acceleration/1(Y)
  Demux/2 -> Velocity/1(Y)
  Demux/1 -> Position/1(Y)
  State/1 -> state2FullState/1
  state2FullState/1 -> Demux/1
  iniVEHposition wrtGLOB [m]/1 -> state2FullState/2
  iniBODYAngles wrtVEH [rad]/1 -> state2FullState/3
  iniVEHAngles wrtGLOB [rad]/1 -> state2FullState/4

== system Collision_two_cars_cs/STATE_BMW_X5_1 ==
  State : Inport  SampleTime=TimeStep
  Acceleration : Subsystem  mask(ToSensorWorld){PortName=Acceleration_BMW_X5_1, PortIndex=21, PortWidth=3, TimeStep=1/20}
      mask prompts: PortName "Port Name [-]"; PortIndex "Index [-]"; PortWidth "Port Dimensions [-]"; TimeStep "Upload Period [s]"
      mask help: Sends signal(s) from Simulink to the Sensor World
      mask Help:
      | Sends signal(s) from Simulink to the Sensor World.
      | 
      | - Port Name [-]: specifies the name of the output terminal of the Simulink block.
      | - Index [-]: specifies the start position in the output vector sent to the Sensor World
      | - Port dimensions [-]: specifies the width (number of scalars) of the output port
      | - Upload period [s]: specifies the upload period (in seconds) of the port.
      mask Display: port_label('input', 1, PortName)
  Demux : Demux  Outputs=5
  Position : Subsystem  mask(ToSensorWorld){PortName=Position_BMW_X5_1, PortIndex=15, PortWidth=3, TimeStep=1/20}
      mask prompts: PortName "Port Name [-]"; PortIndex "Index [-]"; PortWidth "Port Dimensions [-]"; TimeStep "Upload Period [s]"
      mask help: Sends signal(s) from Simulink to the Sensor World
      mask Help:
      | Sends signal(s) from Simulink to the Sensor World.
      | 
      | - Port Name [-]: specifies the name of the output terminal of the Simulink block.
      | - Index [-]: specifies the start position in the output vector sent to the Sensor World
      | - Port dimensions [-]: specifies the width (number of scalars) of the output port
      | - Upload period [s]: specifies the upload period (in seconds) of the port.
      mask Display: port_label('input', 1, PortName)
  RPY : Subsystem  mask(ToSensorWorld){PortName=RPY_BMW_X5_1, PortIndex=24, PortWidth=3, TimeStep=1/20}
      mask prompts: PortName "Port Name [-]"; PortIndex "Index [-]"; PortWidth "Port Dimensions [-]"; TimeStep "Upload Period [s]"
      mask help: Sends signal(s) from Simulink to the Sensor World
      mask Help:
      | Sends signal(s) from Simulink to the Sensor World.
      | 
      | - Port Name [-]: specifies the name of the output terminal of the Simulink block.
      | - Index [-]: specifies the start position in the output vector sent to the Sensor World
      | - Port dimensions [-]: specifies the width (number of scalars) of the output port
      | - Upload period [s]: specifies the upload period (in seconds) of the port.
      mask Display: port_label('input', 1, PortName)
  Velocity : Subsystem  mask(ToSensorWorld){PortName=Velocity_BMW_X5_1, PortIndex=18, PortWidth=3, TimeStep=1/20}
      mask prompts: PortName "Port Name [-]"; PortIndex "Index [-]"; PortWidth "Port Dimensions [-]"; TimeStep "Upload Period [s]"
      mask help: Sends signal(s) from Simulink to the Sensor World
      mask Help:
      | Sends signal(s) from Simulink to the Sensor World.
      | 
      | - Port Name [-]: specifies the name of the output terminal of the Simulink block.
      | - Index [-]: specifies the start position in the output vector sent to the Sensor World
      | - Port dimensions [-]: specifies the width (number of scalars) of the output port
      | - Upload period [s]: specifies the upload period (in seconds) of the port.
      mask Display: port_label('input', 1, PortName)
  iniBODYAngles wrtVEH [rad] : Constant  Value=[Roll0 Pitch0 0]  SampleTime=TimeStep
  iniVEHAngles wrtGLOB [rad] : Constant  Value=[0 0 Yaw0]  SampleTime=TimeStep
  iniVEHposition wrtGLOB [m] : Constant  Value=[x0 y0 z0]  SampleTime=TimeStep
  state2FullState : PreScanSimulinkLibrary/state2FullState  SystemSampleTime=-1
  velRPY : Subsystem  mask(ToSensorWorld){PortName=velRPY_BMW_X5_1, PortIndex=27, PortWidth=3, TimeStep=1/20}
      mask prompts: PortName "Port Name [-]"; PortIndex "Index [-]"; PortWidth "Port Dimensions [-]"; TimeStep "Upload Period [s]"
      mask help: Sends signal(s) from Simulink to the Sensor World
      mask Help:
      | Sends signal(s) from Simulink to the Sensor World.
      | 
      | - Port Name [-]: specifies the name of the output terminal of the Simulink block.
      | - Index [-]: specifies the start position in the output vector sent to the Sensor World
      | - Port dimensions [-]: specifies the width (number of scalars) of the output port
      | - Upload period [s]: specifies the upload period (in seconds) of the port.
      mask Display: port_label('input', 1, PortName)
  wires:
  Demux/5 -> velRPY/1(Y)
  Demux/4 -> RPY/1(Y)
  Demux/3 -> Acceleration/1(Y)
  Demux/2 -> Velocity/1(Y)
  Demux/1 -> Position/1(Y)
  State/1 -> state2FullState/1
  state2FullState/1 -> Demux/1
  iniVEHposition wrtGLOB [m]/1 -> state2FullState/2
  iniBODYAngles wrtVEH [rad]/1 -> state2FullState/3
  iniVEHAngles wrtGLOB [rad]/1 -> state2FullState/4

== system Collision_two_cars_cs/SetActuators ==
  Bus Creator : BusCreator  Inputs=1
  Data Store Read : DataStoreRead  DataStoreName=SimCoreActuators  SampleTime=TimeStep
  SendActuators : M-S-Function  FunctionName=SendActuatorsBlock  Parameters=TimeStep NrOfActuators
  dummy : Outport
  tag scope: SimCoreInfo=global
  wires:
  Bus Creator/1 -> [SimCoreInfo]  "SimCore"
  SendActuators/2 -> Bus Creator/1  "ComputationTime[s]"
  SendActuators/1 -> dummy/1
  Data Store Read/1 -> SendActuators/1

== system Collision_two_cars_cs/SimCoreInfo ==
  Bus Selector : BusSelector  OutputSignals=ComputationTime[s]
  Time : Scope
  wires:
  Bus Selector/1 -> Time/1  "<ComputationTime[s]>"
  [SimCoreInfo] -> Bus Selector/1

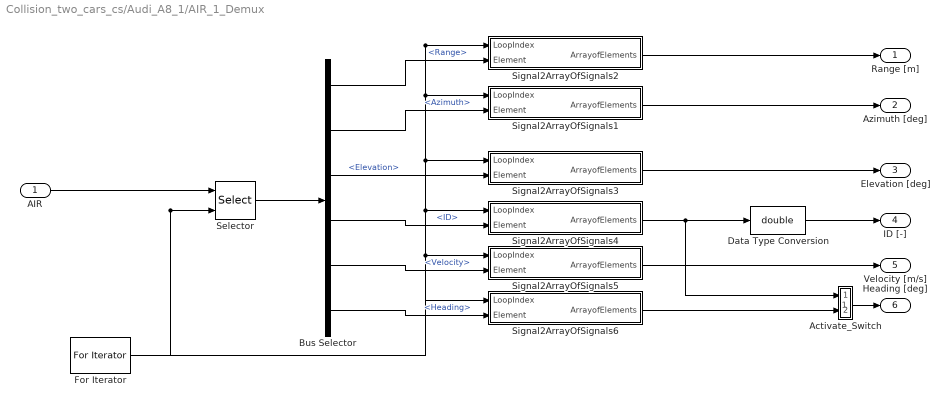
== system Collision_two_cars_cs/Audi_A8_1/AIR_1_Demux ==
  AIR : Inport
  Activate_Switch : Subsystem
      mask Display: text(5,10,'')
  Bus Selector : BusSelector  OutputSignals=DATA.Range,DATA.Azimuth,DATA.Elevation,DATA.ID,DATA.Velocity,DATA.Heading
  Data Type Conversion : DataTypeConversion  OutDataTypeStr=double
  For Iterator : ForIterator  ResetStates=reset  IterationLimit=detectableObjects
  Selector : Selector  InputPortWidth=detectableObjects  IndexOptions=Index vector (port)  Indices=[1 3]  OutputSizes=1
  Signal2ArrayOfSignals1 : Subsystem  mask{VECTORLENGTH=detectableObjects}
      mask prompts: VECTORLENGTH "Length of vector"
  Signal2ArrayOfSignals2 : Subsystem  mask{VECTORLENGTH=detectableObjects}
      mask prompts: VECTORLENGTH "Length of vector"
  Signal2ArrayOfSignals3 : Subsystem  mask{VECTORLENGTH=detectableObjects}
      mask prompts: VECTORLENGTH "Length of vector"
  Signal2ArrayOfSignals4 : Subsystem  mask{VECTORLENGTH=detectableObjects}
      mask prompts: VECTORLENGTH "Length of vector"
  Signal2ArrayOfSignals5 : Subsystem  mask{VECTORLENGTH=detectableObjects}
      mask prompts: VECTORLENGTH "Length of vector"
  Signal2ArrayOfSignals6 : Subsystem  mask{VECTORLENGTH=detectableObjects}
      mask prompts: VECTORLENGTH "Length of vector"
  Range [m] : Outport
  Azimuth [deg] : Outport  Port=2
  Elevation [deg] : Outport  Port=3
  ID [-] : Outport  Port=4
  Velocity [m/s] : Outport  Port=5
  Heading [deg] : Outport  Port=6
  wires:
  Data Type Conversion/1 -> ID [-]/1
  Bus Selector/6 -> Signal2ArrayOfSignals6/2(Element)  "<Heading>"
  Signal2ArrayOfSignals6/1(ArrayofElements) -> Activate_Switch/2(Heading)
  Bus Selector/5 -> Signal2ArrayOfSignals5/2(Element)  "<Velocity>"
  Signal2ArrayOfSignals5/1(ArrayofElements) -> Velocity [m/s]/1
  Bus Selector/4 -> Signal2ArrayOfSignals4/2(Element)  "<ID>"
  Signal2ArrayOfSignals4/1(ArrayofElements) -> Data Type Conversion/1, Activate_Switch/1(BeamID)
  Bus Selector/3 -> Signal2ArrayOfSignals3/2(Element)  "<Elevation>"
  Signal2ArrayOfSignals3/1(ArrayofElements) -> Elevation [deg]/1
  Bus Selector/2 -> Signal2ArrayOfSignals1/2(Element)  "<Azimuth>"
  Signal2ArrayOfSignals1/1(ArrayofElements) -> Azimuth [deg]/1
  Signal2ArrayOfSignals2/1(ArrayofElements) -> Range [m]/1
  Bus Selector/1 -> Signal2ArrayOfSignals2/2(Element)  "<Range>"
  Selector/1 -> Bus Selector/1
  For Iterator/1 -> Signal2ArrayOfSignals6/1(LoopIndex), Signal2ArrayOfSignals5/1(LoopIndex), Signal2ArrayOfSignals4/1(LoopIndex), Signal2ArrayOfSignals3/1(LoopIndex), Signal2ArrayOfSignals1/1(LoopIndex), Signal2ArrayOfSignals2/1(LoopIndex), Selector/2
  AIR/1 -> Selector/1
  Activate_Switch/1(On/Off) -> Heading [deg]/1

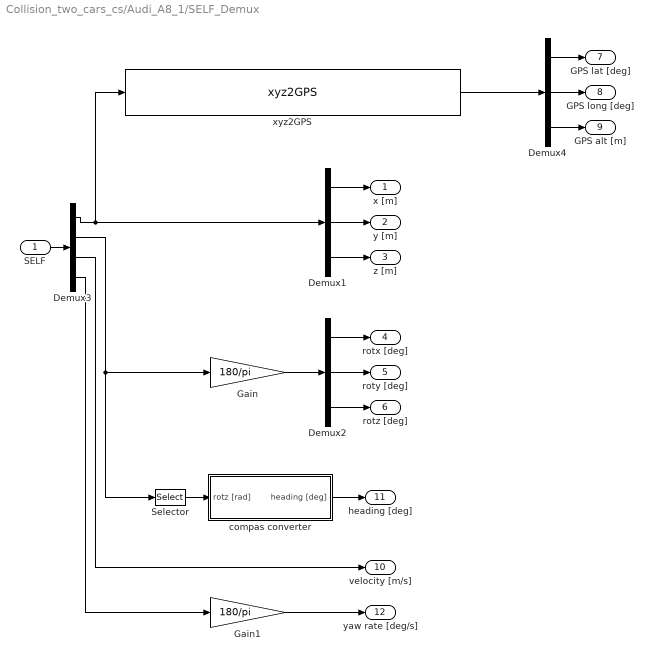
== system Collision_two_cars_cs/Audi_A8_1/SELF_Demux ==
  SELF : Inport
  Demux1 : Demux  Outputs=3
  Demux2 : Demux  Outputs=3
  Demux3 : Demux  Outputs=[3 3 1 1]
  Demux4 : Demux  Outputs=3
  Gain : Gain  Gain=180/pi
  Gain1 : Gain  Gain=180/pi
  Selector : Selector  InputPortWidth=3  IndexOptions=Index vector (dialog)  Indices=[3]  OutputSizes=1
  compas converter : Subsystem
  xyz2GPS : PreScanUsefulBlocks/xyz2GPS  CoordinateCount=1  GPS_base=[48.534599 9.071365 0.000]
  x [m] : Outport
  y [m] : Outport  Port=2
  z [m] : Outport  Port=3
  rotx [deg] : Outport  Port=4
  roty [deg] : Outport  Port=5
  rotz [deg] : Outport  Port=6
  GPS lat [deg] : Outport  Port=7
  GPS long [deg] : Outport  Port=8
  GPS alt [m] : Outport  Port=9
  velocity [m/s] : Outport  Port=10
  heading [deg] : Outport  Port=11
  yaw rate [deg/s] : Outport  Port=12
  wires:
  Demux3/4 -> Gain1/1
  Gain1/1 -> yaw rate [deg/s]/1
  Demux3/3 -> velocity [m/s]/1
  compas converter/1(heading [deg]) -> heading [deg]/1
  xyz2GPS/1 -> Demux4/1
  Demux4/3 -> GPS alt [m]/1
  Demux4/2 -> GPS long [deg]/1
  Demux4/1 -> GPS lat [deg]/1
  Demux3/2 -> Gain/1, Selector/1
  Demux3/1 -> xyz2GPS/1, Demux1/1
  SELF/1 -> Demux3/1
  Demux2/3 -> rotz [deg]/1
  Demux2/2 -> roty [deg]/1
  Demux2/1 -> rotx [deg]/1
  Demux1/3 -> z [m]/1
  Demux1/2 -> y [m]/1
  Demux1/1 -> x [m]/1
  Gain/1 -> Demux2/1
  Selector/1 -> compas converter/1(rotz [rad])

== system Collision_two_cars_cs/Audi_A8_1/Trajectories ==
  Traj2State1 : Subsystem  Tag=Traj2State  mask(PreScan Demux Block:){}
      settings: DeleteFcn=PreScanBlockDeleteFcn;
  Trajectory_1 : Subsystem  Tag=Trajectory  mask(PreScan Source Block: Trajectory){FileName='Trajectory_1_Synced.mat', TimeStep=1/20}
      mask prompts: TimeStep "Time Step [s]"
      mask help:
      | The Trajectory block contains the trajectories defined in the PreScan Experiment Editor. The output of the trajectory block is the (vehicle) State.
      |
      | For more information, please click Help.
      mask init:
      | [direc,name]=fileparts(get_param(bdroot, 'FileName'));
      | load([direc,'/Trajectories/',FileName])
      | trajectory=trajectory';
      | 
      | traj.time=trajectory(:,1);%[];
      | traj.signals.values=trajectory(:,2:19);
      | traj.dimensions=18;
      | traj.label='';
      | 
      | SampleTime=traj.time(2)-traj.time(1);
      settings: DeleteFcn=PreScanBlockDeleteFcn;
      mask Help: eval('openHelp(312)')
      mask Display: fprintf(FileName)
  Trajectory_1_Offset : Constant  Tag=TrajectoryOffset  Value="[0  0  0  0  0  0]"
  State : Outport  Tag=TrajOutport
  wires:
  Trajectory_1/1(trajectory) -> Traj2State1/1(Traj Org)
  Trajectory_1_Offset/1 -> Traj2State1/2(Offset)
  Traj2State1/1(state) -> State/1

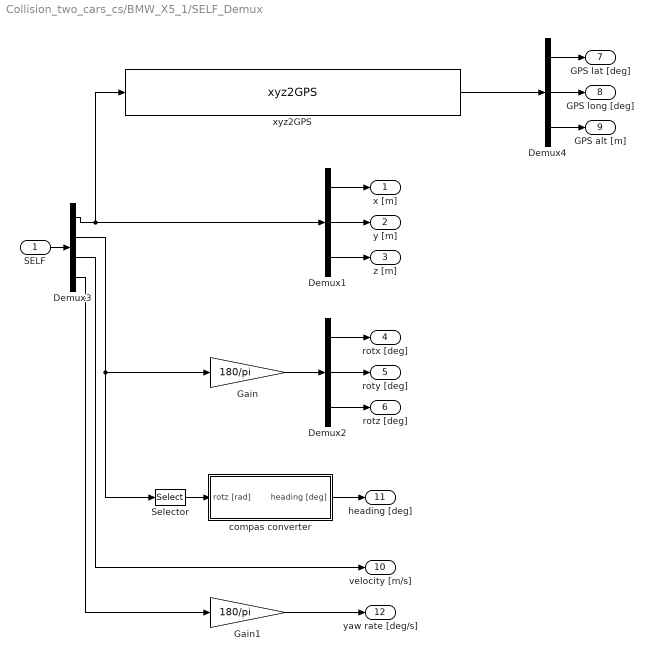
== system Collision_two_cars_cs/BMW_X5_1/SELF_Demux ==
  SELF : Inport
  Demux1 : Demux  Outputs=3
  Demux2 : Demux  Outputs=3
  Demux3 : Demux  Outputs=[3 3 1 1]
  Demux4 : Demux  Outputs=3
  Gain : Gain  Gain=180/pi
  Gain1 : Gain  Gain=180/pi
  Selector : Selector  InputPortWidth=3  IndexOptions=Index vector (dialog)  Indices=[3]  OutputSizes=1
  compas converter : Subsystem
  xyz2GPS : PreScanUsefulBlocks/xyz2GPS  CoordinateCount=1  GPS_base=[48.534599 9.071365 0.000]
  x [m] : Outport
  y [m] : Outport  Port=2
  z [m] : Outport  Port=3
  rotx [deg] : Outport  Port=4
  roty [deg] : Outport  Port=5
  rotz [deg] : Outport  Port=6
  GPS lat [deg] : Outport  Port=7
  GPS long [deg] : Outport  Port=8
  GPS alt [m] : Outport  Port=9
  velocity [m/s] : Outport  Port=10
  heading [deg] : Outport  Port=11
  yaw rate [deg/s] : Outport  Port=12
  wires:
  Demux3/4 -> Gain1/1
  Gain1/1 -> yaw rate [deg/s]/1
  Demux3/3 -> velocity [m/s]/1
  compas converter/1(heading [deg]) -> heading [deg]/1
  xyz2GPS/1 -> Demux4/1
  Demux4/3 -> GPS alt [m]/1
  Demux4/2 -> GPS long [deg]/1
  Demux4/1 -> GPS lat [deg]/1
  Demux3/2 -> Gain/1, Selector/1
  Demux3/1 -> xyz2GPS/1, Demux1/1
  SELF/1 -> Demux3/1
  Demux2/3 -> rotz [deg]/1
  Demux2/2 -> roty [deg]/1
  Demux2/1 -> rotx [deg]/1
  Demux1/3 -> z [m]/1
  Demux1/2 -> y [m]/1
  Demux1/1 -> x [m]/1
  Gain/1 -> Demux2/1
  Selector/1 -> compas converter/1(rotz [rad])

== system Collision_two_cars_cs/BMW_X5_1/Trajectories ==
  Traj2State1 : Subsystem  Tag=Traj2State  mask(PreScan Demux Block:){}
      settings: DeleteFcn=PreScanBlockDeleteFcn;
  Trajectory_2 : Subsystem  Tag=Trajectory  mask(PreScan Source Block: Trajectory){FileName='Trajectory_2_Synced.mat', TimeStep=1/20}
      mask prompts: TimeStep "Time Step [s]"
      mask help:
      | The Trajectory block contains the trajectories defined in the PreScan Experiment Editor. The output of the trajectory block is the (vehicle) State.
      |
      | For more information, please click Help.
      mask init: same as Collision_two_cars_cs/Audi_A8_1/Trajectories/Trajectory_1
      settings: DeleteFcn=PreScanBlockDeleteFcn;
      mask Help: eval('openHelp(312)')
      mask Display: fprintf(FileName)
  Trajectory_2_Offset : Constant  Tag=TrajectoryOffset  Value="[0  0  0  0  0  0]"
  State : Outport  Tag=TrajOutport
  wires:
  Trajectory_2/1(trajectory) -> Traj2State1/1(Traj Org)
  Trajectory_2_Offset/1 -> Traj2State1/2(Offset)
  Traj2State1/1(state) -> State/1

== system Collision_two_cars_cs/STATE_Audi_A8_1/Acceleration ==
  Y : Inport
  Assignment : Assignment  IndexMode=Zero-based  SampleTime=TimeStep  IndexOptions=Starting index (dialog)  Indices=PortIndex  OutputSizes=[1 1]
  Data Store Read : DataStoreRead  DataStoreName=SimCoreActuators  SampleTime=TimeStep
  Data Store Write : DataStoreWrite  DataStoreName=SimCoreActuators
  wires:
  Assignment/1 -> Data Store Write/1
  Data Store Read/1 -> Assignment/1
  Y/1 -> Assignment/2

== system Collision_two_cars_cs/STATE_Audi_A8_1/Position ==
  Y : Inport
  Assignment : Assignment  IndexMode=Zero-based  SampleTime=TimeStep  IndexOptions=Starting index (dialog)  Indices=PortIndex  OutputSizes=[1 1]
  Data Store Read : DataStoreRead  DataStoreName=SimCoreActuators  SampleTime=TimeStep
  Data Store Write : DataStoreWrite  DataStoreName=SimCoreActuators
  wires:
  Y/1 -> Assignment/2
  Data Store Read/1 -> Assignment/1
  Assignment/1 -> Data Store Write/1

== system Collision_two_cars_cs/STATE_Audi_A8_1/RPY ==
  Y : Inport
  Assignment : Assignment  IndexMode=Zero-based  SampleTime=TimeStep  IndexOptions=Starting index (dialog)  Indices=PortIndex  OutputSizes=[1 1]
  Data Store Read : DataStoreRead  DataStoreName=SimCoreActuators  SampleTime=TimeStep
  Data Store Write : DataStoreWrite  DataStoreName=SimCoreActuators
  wires:
  Assignment/1 -> Data Store Write/1
  Data Store Read/1 -> Assignment/1
  Y/1 -> Assignment/2

== system Collision_two_cars_cs/STATE_Audi_A8_1/Velocity ==
  Y : Inport
  Assignment : Assignment  IndexMode=Zero-based  SampleTime=TimeStep  IndexOptions=Starting index (dialog)  Indices=PortIndex  OutputSizes=[1 1]
  Data Store Read : DataStoreRead  DataStoreName=SimCoreActuators  SampleTime=TimeStep
  Data Store Write : DataStoreWrite  DataStoreName=SimCoreActuators
  wires:
  Assignment/1 -> Data Store Write/1
  Data Store Read/1 -> Assignment/1
  Y/1 -> Assignment/2

== system Collision_two_cars_cs/STATE_Audi_A8_1/velRPY ==
  Y : Inport
  Assignment : Assignment  IndexMode=Zero-based  SampleTime=TimeStep  IndexOptions=Starting index (dialog)  Indices=PortIndex  OutputSizes=[1 1]
  Data Store Read : DataStoreRead  DataStoreName=SimCoreActuators  SampleTime=TimeStep
  Data Store Write : DataStoreWrite  DataStoreName=SimCoreActuators
  wires:
  Assignment/1 -> Data Store Write/1
  Data Store Read/1 -> Assignment/1
  Y/1 -> Assignment/2

== system Collision_two_cars_cs/STATE_BMW_X5_1/Acceleration ==
  Y : Inport
  Assignment : Assignment  IndexMode=Zero-based  SampleTime=TimeStep  IndexOptions=Starting index (dialog)  Indices=PortIndex  OutputSizes=[1 1]
  Data Store Read : DataStoreRead  DataStoreName=SimCoreActuators  SampleTime=TimeStep
  Data Store Write : DataStoreWrite  DataStoreName=SimCoreActuators
  wires:
  Assignment/1 -> Data Store Write/1
  Data Store Read/1 -> Assignment/1
  Y/1 -> Assignment/2

== system Collision_two_cars_cs/STATE_BMW_X5_1/Position ==
  Y : Inport
  Assignment : Assignment  IndexMode=Zero-based  SampleTime=TimeStep  IndexOptions=Starting index (dialog)  Indices=PortIndex  OutputSizes=[1 1]
  Data Store Read : DataStoreRead  DataStoreName=SimCoreActuators  SampleTime=TimeStep
  Data Store Write : DataStoreWrite  DataStoreName=SimCoreActuators
  wires:
  Y/1 -> Assignment/2
  Data Store Read/1 -> Assignment/1
  Assignment/1 -> Data Store Write/1

== system Collision_two_cars_cs/STATE_BMW_X5_1/RPY ==
  Y : Inport
  Assignment : Assignment  IndexMode=Zero-based  SampleTime=TimeStep  IndexOptions=Starting index (dialog)  Indices=PortIndex  OutputSizes=[1 1]
  Data Store Read : DataStoreRead  DataStoreName=SimCoreActuators  SampleTime=TimeStep
  Data Store Write : DataStoreWrite  DataStoreName=SimCoreActuators
  wires:
  Assignment/1 -> Data Store Write/1
  Data Store Read/1 -> Assignment/1
  Y/1 -> Assignment/2

== system Collision_two_cars_cs/STATE_BMW_X5_1/Velocity ==
  Y : Inport
  Assignment : Assignment  IndexMode=Zero-based  SampleTime=TimeStep  IndexOptions=Starting index (dialog)  Indices=PortIndex  OutputSizes=[1 1]
  Data Store Read : DataStoreRead  DataStoreName=SimCoreActuators  SampleTime=TimeStep
  Data Store Write : DataStoreWrite  DataStoreName=SimCoreActuators
  wires:
  Assignment/1 -> Data Store Write/1
  Data Store Read/1 -> Assignment/1
  Y/1 -> Assignment/2

== system Collision_two_cars_cs/STATE_BMW_X5_1/velRPY ==
  Y : Inport
  Assignment : Assignment  IndexMode=Zero-based  SampleTime=TimeStep  IndexOptions=Starting index (dialog)  Indices=PortIndex  OutputSizes=[1 1]
  Data Store Read : DataStoreRead  DataStoreName=SimCoreActuators  SampleTime=TimeStep
  Data Store Write : DataStoreWrite  DataStoreName=SimCoreActuators
  wires:
  Assignment/1 -> Data Store Write/1
  Data Store Read/1 -> Assignment/1
  Y/1 -> Assignment/2

== system Collision_two_cars_cs/Audi_A8_1/AIR_1_Demux/Activate_Switch ==
  BeamID : Inport
  Heading : Inport  Port=2
  Constant : Constant  Value=0
  Product1 : Product  RndMeth=Zero
  Relational Operator : RelationalOperator  Operator=~=  OutDataTypeStr=boolean
  On/Off : Outport
  wires:
  Constant/1 -> Relational Operator/1
  Relational Operator/1 -> Product1/1
  BeamID/1 -> Relational Operator/2
  Product1/1 -> On/Off/1
  Heading/1 -> Product1/2

== system Collision_two_cars_cs/Audi_A8_1/AIR_1_Demux/Signal2ArrayOfSignals1 ==
  note: Set mask parameter VECTORLENGTH
      |  to MAXMESSAGES
  note: Initial state of Previous vector block
      | set to zeros(VECTORLENGTH,1)
  LoopIndex : Inport
  Element : Inport  Port=2
  Assignment : Assignment  IndexOptions=Index vector (port)  Indices=1  OutputSizes=1
  Previous vector : Memory  X0=zeros(VECTORLENGTH,1)  InheritSampleTime=on
  ArrayofElements : Outport
  wires:
  Element/1 -> Assignment/2
  LoopIndex/1 -> Assignment/3
  Previous vector/1 -> Assignment/1
  Assignment/1 -> ArrayofElements/1, Previous vector/1

== system Collision_two_cars_cs/Audi_A8_1/AIR_1_Demux/Signal2ArrayOfSignals2 ==
  note: Set mask parameter VECTORLENGTH
      |  to MAXMESSAGES
  note: Initial state of Previous vector block
      | set to zeros(VECTORLENGTH,1)
  LoopIndex : Inport
  Element : Inport  Port=2
  Assignment : Assignment  IndexOptions=Index vector (port)  Indices=1  OutputSizes=1
  Previous vector : Memory  X0=zeros(VECTORLENGTH,1)  InheritSampleTime=on
  ArrayofElements : Outport
  wires:
  Element/1 -> Assignment/2
  LoopIndex/1 -> Assignment/3
  Previous vector/1 -> Assignment/1
  Assignment/1 -> ArrayofElements/1, Previous vector/1

== system Collision_two_cars_cs/Audi_A8_1/AIR_1_Demux/Signal2ArrayOfSignals3 ==
  note: Set mask parameter VECTORLENGTH
      |  to MAXMESSAGES
  note: Initial state of Previous vector block
      | set to zeros(VECTORLENGTH,1)
  LoopIndex : Inport
  Element : Inport  Port=2
  Assignment : Assignment  IndexOptions=Index vector (port)  Indices=1  OutputSizes=1
  Previous vector : Memory  X0=zeros(VECTORLENGTH,1)  InheritSampleTime=on
  ArrayofElements : Outport
  wires:
  Element/1 -> Assignment/2
  LoopIndex/1 -> Assignment/3
  Previous vector/1 -> Assignment/1
  Assignment/1 -> ArrayofElements/1, Previous vector/1

== system Collision_two_cars_cs/Audi_A8_1/AIR_1_Demux/Signal2ArrayOfSignals4 ==
  note: Set mask parameter VECTORLENGTH
      |  to MAXMESSAGES
  note: Initial state of Previous vector block
      | set to zeros(VECTORLENGTH,1)
  LoopIndex : Inport
  Element : Inport  Port=2
  Assignment : Assignment  IndexOptions=Index vector (port)  Indices=1  OutputSizes=1
  Previous vector : Memory  X0=zeros(VECTORLENGTH,1)  InheritSampleTime=on
  ArrayofElements : Outport
  wires:
  Element/1 -> Assignment/2
  LoopIndex/1 -> Assignment/3
  Previous vector/1 -> Assignment/1
  Assignment/1 -> ArrayofElements/1, Previous vector/1

== system Collision_two_cars_cs/Audi_A8_1/AIR_1_Demux/Signal2ArrayOfSignals5 ==
  note: Set mask parameter VECTORLENGTH
      |  to MAXMESSAGES
  note: Initial state of Previous vector block
      | set to zeros(VECTORLENGTH,1)
  LoopIndex : Inport
  Element : Inport  Port=2
  Assignment : Assignment  IndexOptions=Index vector (port)  Indices=1  OutputSizes=1
  Previous vector : Memory  X0=zeros(VECTORLENGTH,1)  InheritSampleTime=on
  ArrayofElements : Outport
  wires:
  Element/1 -> Assignment/2
  LoopIndex/1 -> Assignment/3
  Previous vector/1 -> Assignment/1
  Assignment/1 -> ArrayofElements/1, Previous vector/1

== system Collision_two_cars_cs/Audi_A8_1/AIR_1_Demux/Signal2ArrayOfSignals6 ==
  note: Set mask parameter VECTORLENGTH
      |  to MAXMESSAGES
  note: Initial state of Previous vector block
      | set to zeros(VECTORLENGTH,1)
  LoopIndex : Inport
  Element : Inport  Port=2
  Assignment : Assignment  IndexOptions=Index vector (port)  Indices=1  OutputSizes=1
  Previous vector : Memory  X0=zeros(VECTORLENGTH,1)  InheritSampleTime=on
  ArrayofElements : Outport
  wires:
  Element/1 -> Assignment/2
  LoopIndex/1 -> Assignment/3
  Previous vector/1 -> Assignment/1
  Assignment/1 -> ArrayofElements/1, Previous vector/1

== system Collision_two_cars_cs/Audi_A8_1/SELF_Demux/compas converter ==
  rotz [rad] : Inport
  cart2compas : Subsystem
  rad2deg : Gain  Gain=180/pi
  heading [deg] : Outport
  wires:
  cart2compas/1(heading [deg]) -> heading [deg]/1
  rotz [rad]/1 -> rad2deg/1
  rad2deg/1 -> cart2compas/1(Angle [deg])

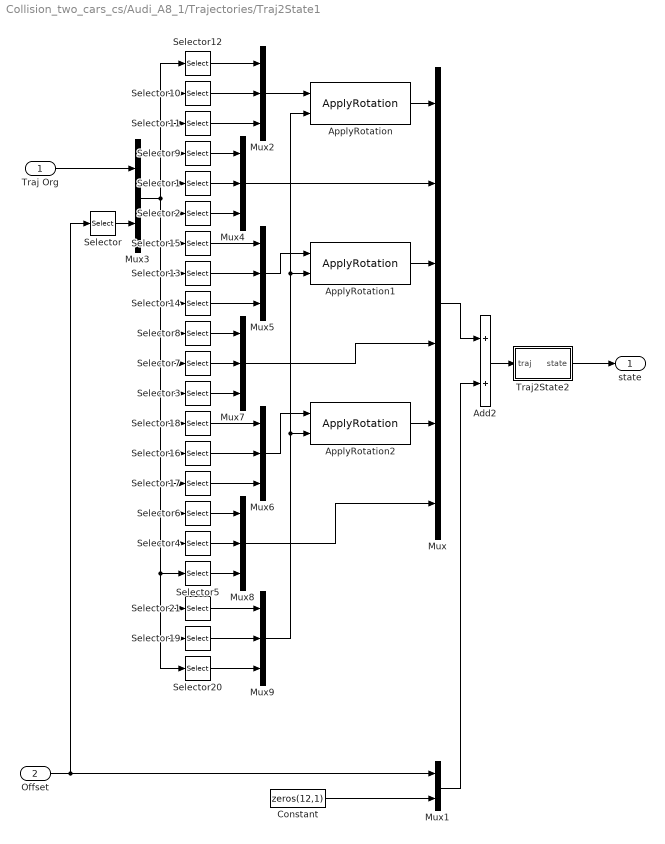
== system Collision_two_cars_cs/Audi_A8_1/Trajectories/Traj2State1 ==
  Traj Org : Inport
  Offset : Inport  Port=2
  Add2 : Sum
  ApplyRotation : PreScanSimulinkLibrary/ApplyRotation
  ApplyRotation1 : PreScanSimulinkLibrary/ApplyRotation
  ApplyRotation2 : PreScanSimulinkLibrary/ApplyRotation
  Constant : Constant  Value=zeros(12,1)
  Mux : Mux  Inputs=6
  Mux1 : Mux  Inputs=2
  Mux{2,4..9} (7 alike) : Mux  Inputs=3
  Mux3 : Mux  Inputs=2
  Selector : Selector  InputPortWidth=6  IndexOptions=Index vector (dialog)  Indices=[4 5 6]  OutputSizes=1
  Selector1 : Selector  InputPortWidth=21  IndexOptions=Index vector (dialog)  Indices=[5]  OutputSizes=1
  Selector10 : Selector  InputPortWidth=21  IndexOptions=Index vector (dialog)  Indices=[2]  OutputSizes=1
  Selector11 : Selector  InputPortWidth=21  IndexOptions=Index vector (dialog)  Indices=[3]  OutputSizes=1
  Selector12 : Selector  InputPortWidth=21  IndexOptions=Index vector (dialog)  Indices=[1]  OutputSizes=1
  Selector13 : Selector  InputPortWidth=21  IndexOptions=Index vector (dialog)  Indices=[8]  OutputSizes=1
  Selector14 : Selector  InputPortWidth=21  IndexOptions=Index vector (dialog)  Indices=[9]  OutputSizes=1
  Selector15 : Selector  InputPortWidth=21  IndexOptions=Index vector (dialog)  Indices=[7]  OutputSizes=1
  Selector16 : Selector  InputPortWidth=21  IndexOptions=Index vector (dialog)  Indices=[14]  OutputSizes=1
  Selector17 : Selector  InputPortWidth=21  IndexOptions=Index vector (dialog)  Indices=[15]  OutputSizes=1
  Selector18 : Selector  InputPortWidth=21  IndexOptions=Index vector (dialog)  Indices=[13]  OutputSizes=1
  Selector19 : Selector  InputPortWidth=21  IndexOptions=Index vector (dialog)  Indices=[20]  OutputSizes=1
  Selector2 : Selector  InputPortWidth=21  IndexOptions=Index vector (dialog)  Indices=[6]  OutputSizes=1
  Selector20 : Selector  InputPortWidth=21  IndexOptions=Index vector (dialog)  Indices=[21]  OutputSizes=1
  Selector21 : Selector  InputPortWidth=21  IndexOptions=Index vector (dialog)  Indices=[19]  OutputSizes=1
  Selector3 : Selector  InputPortWidth=21  IndexOptions=Index vector (dialog)  Indices=[12]  OutputSizes=1
  Selector4 : Selector  InputPortWidth=21  IndexOptions=Index vector (dialog)  Indices=[17]  OutputSizes=1
  Selector5 : Selector  InputPortWidth=21  IndexOptions=Index vector (dialog)  Indices=[18]  OutputSizes=1
  Selector6 : Selector  InputPortWidth=21  IndexOptions=Index vector (dialog)  Indices=[16]  OutputSizes=1
  Selector7 : Selector  InputPortWidth=21  IndexOptions=Index vector (dialog)  Indices=[11]  OutputSizes=1
  Selector8 : Selector  InputPortWidth=21  IndexOptions=Index vector (dialog)  Indices=[10]  OutputSizes=1
  Selector9 : Selector  InputPortWidth=21  IndexOptions=Index vector (dialog)  Indices=[4]  OutputSizes=1
  Traj2State2 : Subsystem
  state : Outport
  wires:
  Mux9/1 -> ApplyRotation2/2, ApplyRotation1/2, ApplyRotation/2
  Selector20/1 -> Mux9/3
  Selector19/1 -> Mux9/2
  Selector21/1 -> Mux9/1
  Selector5/1 -> Mux8/3
  Selector4/1 -> Mux8/2
  Selector6/1 -> Mux8/1
  Mux8/1 -> Mux/6
  Mux6/1 -> ApplyRotation2/1
  Mux7/1 -> Mux/4
  ApplyRotation2/1 -> Mux/5
  Selector3/1 -> Mux7/3
  Selector7/1 -> Mux7/2
  Selector8/1 -> Mux7/1
  Mux4/1 -> Mux/2
  Mux5/1 -> ApplyRotation1/1
  ApplyRotation1/1 -> Mux/3
  Mux2/1 -> ApplyRotation/1
  ApplyRotation/1 -> Mux/1
  Selector2/1 -> Mux4/3
  Selector1/1 -> Mux4/2
  Selector9/1 -> Mux4/1
  Selector17/1 -> Mux6/3
  Selector16/1 -> Mux6/2
  Selector18/1 -> Mux6/1
  Selector14/1 -> Mux5/3
  Selector13/1 -> Mux5/2
  Selector15/1 -> Mux5/1
  Selector11/1 -> Mux2/3
  Selector10/1 -> Mux2/2
  Selector12/1 -> Mux2/1
  Mux3/1 -> Selector8/1, Selector7/1, Selector3/1, Selector18/1, Selector16/1, Selector17/1, Selector6/1, Selector20/1, Selector19/1, Selector21/1, Selector5/1, Selector4/1, Selector14/1, Selector13/1, Selector15/1, Selector2/1, Selector1/1, Selector9/1, Selector12/1, Selector10/1, Selector11/1
  Mux1/1 -> Add2/2
  Constant/1 -> Mux1/2
  Add2/1 -> Traj2State2/1(traj)
  Selector/1 -> Mux3/2
  Traj Org/1 -> Mux3/1
  Offset/1 -> Mux1/1, Selector/1
  Mux/1 -> Add2/1
  Traj2State2/1(state) -> state/1

== system Collision_two_cars_cs/Audi_A8_1/Trajectories/Trajectory_1 ==
  From Workspace : FromWorkspace  VariableName=trajectory  SampleTime=TimeStep  OutputAfterFinalValue=Holding final value
  From Workspace1 : FromWorkspace  VariableName=trajectory  SampleTime=TimeStep  OutputAfterFinalValue=Setting to zero
  Mux : Mux  Inputs=2
  Selector1 : Selector  InputPortWidth=24  IndexOptions=Index vector (dialog)  Indices=[7:18]  OutputSizes=1
  Selector9 : Selector  InputPortWidth=24  IndexOptions=Index vector (dialog)  Indices=[1:6]  OutputSizes=1
  trajectory : Outport
  wires:
  Selector1/1 -> Mux/2
  Selector9/1 -> Mux/1
  Mux/1 -> trajectory/1
  From Workspace1/1 -> Selector1/1
  From Workspace/1 -> Selector9/1

== system Collision_two_cars_cs/BMW_X5_1/SELF_Demux/compas converter ==
  rotz [rad] : Inport
  cart2compas : Subsystem
  rad2deg : Gain  Gain=180/pi
  heading [deg] : Outport
  wires:
  cart2compas/1(heading [deg]) -> heading [deg]/1
  rotz [rad]/1 -> rad2deg/1
  rad2deg/1 -> cart2compas/1(Angle [deg])
